simulink model "Simple_2Quad_payload_01"  (R2018b)
settings: Solver=VariableStepAuto  StartTime=0.0  StopTime=40  RelTol=1e-3
InitFcn:
  | Simple_2Quad_payload_01_const
values from neighbouring files (symbols this model uses):
  d = 1    [Simple_2Quad_payload_01_const.m]    (also in Simple_2Quad_payload_02_const.m; Simple_2Quad_payload_03_const.m; Simple_2Quad_payload_04_const.m)
  g = 9.81    [Colab_4Quad_model_01_const.m]    (also in Colab_4Quad_model_02_const.m; Simple_2Quad_payload_01_const.m; Simple_2Quad_payload_02_const.m; Simple_2Quad_payload_03_const.m)
  I = 1    [Simple_2Quad_payload_01_const.m]    (also in Simple_2Quad_payload_02_const.m; Simple_2Quad_payload_03_const.m; Simple_2Quad_payload_04_const.m)
  l2 = 1    [Simple_2Quad_payload_01_const.m]    (also in Simple_2Quad_payload_02_const.m; Simple_2Quad_payload_03_const.m)
  M = 1.0    (= 1)    [Colab_4Quad_model_01_const.m]    (also in Colab_4Quad_model_02_const.m; Simple_2Quad_payload_01_const.m; Simple_2Quad_payload_02_const.m; Simple_2Quad_payload_03_const.m)
  m1 = 1    [Simple_2Quad_payload_01_const.m]    (also in Simple_2Quad_payload_02_const.m; Simple_2Quad_payload_03_const.m)
  m2 = 1    [Simple_2Quad_payload_01_const.m]    (also in Simple_2Quad_payload_02_const.m; Simple_2Quad_payload_03_const.m)
settings Model: Creator=ali  LastModifiedBy=ali

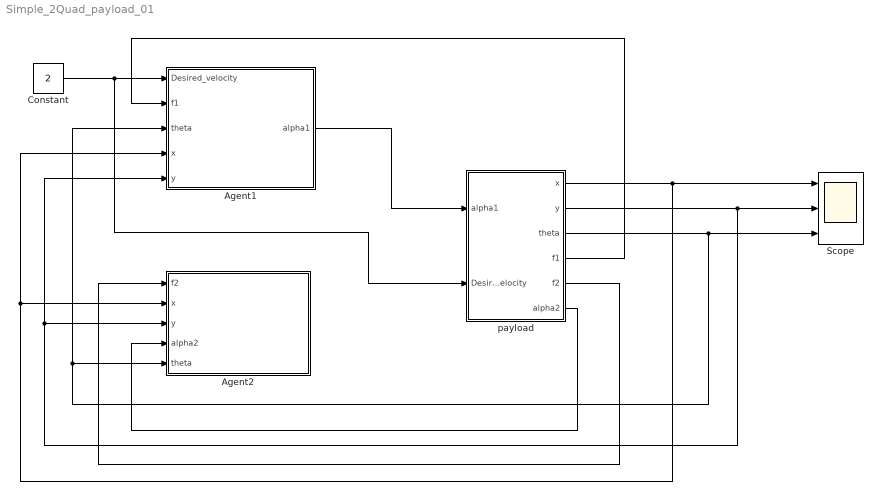
== system Simple_2Quad_payload_01 ==
  Agent1 : Subsystem
  Agent2 : Subsystem
  Constant : Constant  Value=2
  Scope : Scope  NumInputPorts=3
  payload : Subsystem
  wires:
  Constant/1 -> payload/2(Desired_velocity), Agent1/1(Desired_velocity)
  payload/3(theta) -> Scope/3, Agent2/5(theta), Agent1/3(theta)
  payload/1(x) -> Scope/1, Agent2/2(x), Agent1/4(x)
  payload/2(y) -> Scope/2, Agent2/3(y), Agent1/5(y)
  Agent1/1(alpha1) -> payload/1(alpha1)
  payload/4(f1) -> Agent1/2(f1)
  payload/5(f2) -> Agent2/1(f2)
  payload/6(alpha2) -> Agent2/4(alpha2)

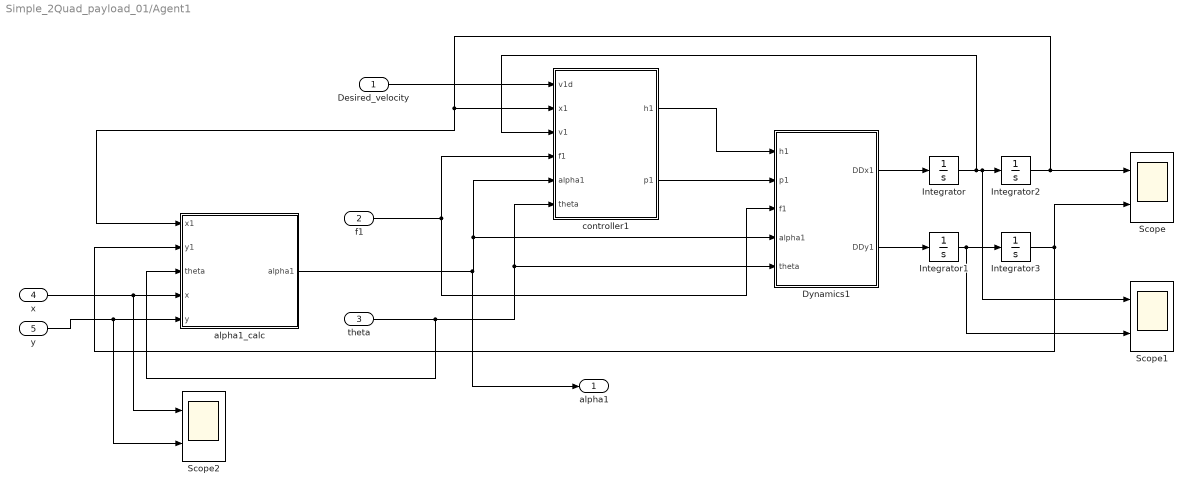
== system Simple_2Quad_payload_01/Agent1 ==
  Desired_velocity : Inport
  f1 : Inport  Port=2
  theta : Inport  Port=3
  x : Inport  Port=4
  y : Inport  Port=5
  Dynamics1 : MATLAB Function  TreatAsAtomicUnit=on
  Integrator : Integrator
  Integrator1 : Integrator
  Integrator2 : Integrator  InitialCondition=1
  Integrator3 : Integrator  InitialCondition=10
  Scope : Scope  NumInputPorts=2
  Scope1 : Scope  NumInputPorts=2
  Scope2 : Scope  NumInputPorts=2
  alpha1_calc : MATLAB Function  TreatAsAtomicUnit=on
  controller1 : Subsystem
  alpha1 : Outport
  wires:
  Dynamics1/1(DDx1) -> Integrator/1
  Dynamics1/2(DDy1) -> Integrator1/1
  Integrator/1 -> Scope1/1, Integrator2/1, controller1/3(v1)
  Integrator1/1 -> Scope1/2, Integrator3/1
  Integrator2/1 -> Scope/1, controller1/2(x1), alpha1_calc/1(x1)
  Integrator3/1 -> alpha1_calc/2(y1), Scope/2
  controller1/2(p1) -> Dynamics1/2(p1)
  controller1/1(h1) -> Dynamics1/1(h1)
  Desired_velocity/1 -> controller1/1(v1d)
  f1/1 -> controller1/4(f1), Dynamics1/3(f1)
  alpha1_calc/1(alpha1) -> alpha1/1, controller1/5(alpha1), Dynamics1/4(alpha1)
  theta/1 -> alpha1_calc/3(theta), Dynamics1/5(theta), controller1/6(theta)
  x/1 -> Scope2/1, alpha1_calc/4(x)
  y/1 -> Scope2/2, alpha1_calc/5(y)

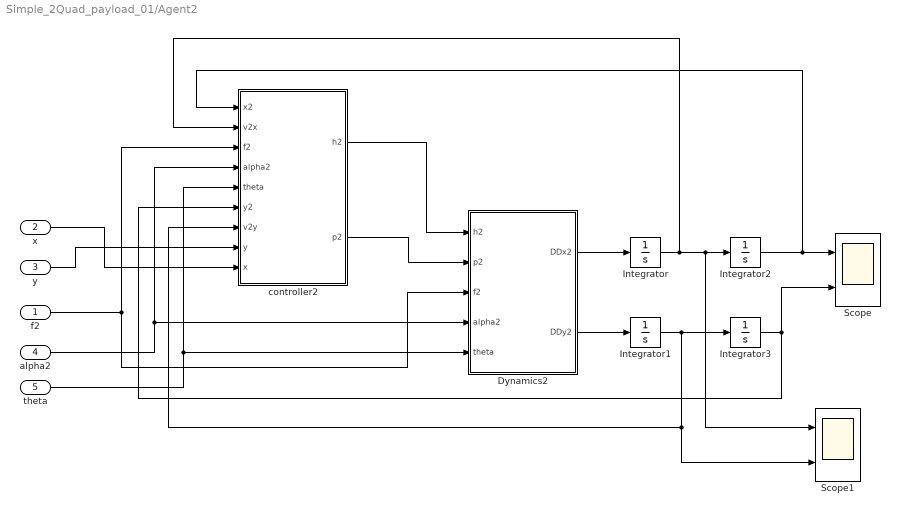
== system Simple_2Quad_payload_01/Agent2 ==
  f2 : Inport
  x : Inport  Port=2
  y : Inport  Port=3
  alpha2 : Inport  Port=4
  theta : Inport  Port=5
  Dynamics2 : MATLAB Function  TreatAsAtomicUnit=on
  Integrator : Integrator
  Integrator1 : Integrator
  Integrator2 : Integrator  InitialCondition=-1
  Integrator3 : Integrator  InitialCondition=10
  Scope : Scope  NumInputPorts=2
  Scope1 : Scope  NumInputPorts=2
  controller2 : Subsystem
  wires:
  theta/1 -> controller2/5(theta), Dynamics2/5(theta)
  alpha2/1 -> controller2/4(alpha2), Dynamics2/4(alpha2)
  f2/1 -> Dynamics2/3(f2), controller2/3(f2)
  controller2/1(h2) -> Dynamics2/1(h2)
  controller2/2(p2) -> Dynamics2/2(p2)
  Integrator3/1 -> controller2/6(y2), Scope/2
  Integrator2/1 -> controller2/1(x2), Scope/1
  Integrator1/1 -> Scope1/2, controller2/7(v2y), Integrator3/1
  Integrator/1 -> controller2/2(v2x), Scope1/1, Integrator2/1
  Dynamics2/2(DDy2) -> Integrator1/1
  Dynamics2/1(DDx2) -> Integrator/1
  y/1 -> controller2/8(y)
  x/1 -> controller2/9(x)

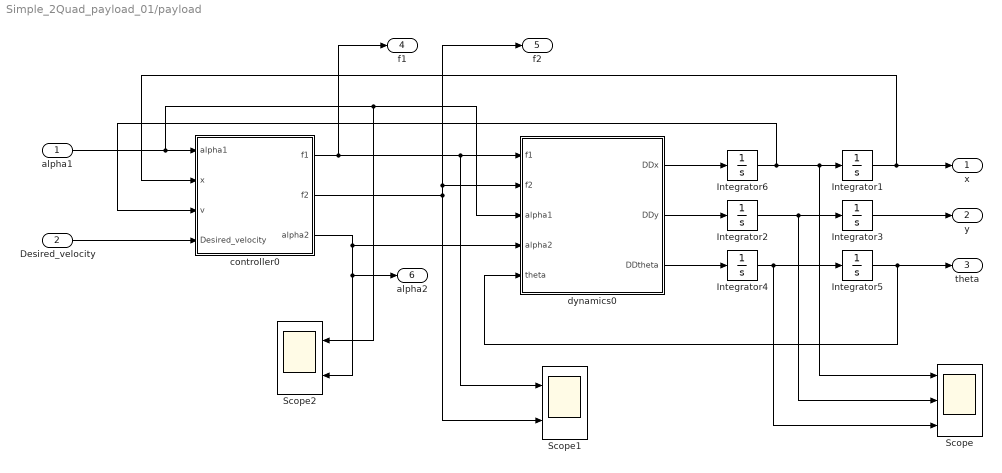
== system Simple_2Quad_payload_01/payload ==
  alpha1 : Inport
  Desired_velocity : Inport  Port=2
  Integrator{1..2,4..6} (5 alike) : Integrator
  Integrator3 : Integrator  InitialCondition=9
  Scope : Scope  NumInputPorts=3
  Scope1 : Scope  NumInputPorts=2
  Scope2 : Scope  NumInputPorts=2
  controller0 : Subsystem
  dynamics0 : MATLAB Function  TreatAsAtomicUnit=on
  x : Outport
  y : Outport  Port=2
  theta : Outport  Port=3
  f1 : Outport  Port=4
  f2 : Outport  Port=5
  alpha2 : Outport  Port=6
  wires:
  dynamics0/1(DDx) -> Integrator6/1
  dynamics0/2(DDy) -> Integrator2/1
  dynamics0/3(DDtheta) -> Integrator4/1
  Integrator4/1 -> Scope/3, Integrator5/1
  Integrator1/1 -> controller0/2(x), x/1
  Integrator3/1 -> y/1
  Integrator5/1 -> dynamics0/5(theta), theta/1
  controller0/1(f1) -> f1/1, dynamics0/1(f1), Scope1/1
  controller0/2(f2) -> f2/1, dynamics0/2(f2), Scope1/2
  controller0/3(alpha2) -> Scope2/2, alpha2/1, dynamics0/4(alpha2)
  alpha1/1 -> dynamics0/3(alpha1), Scope2/1, controller0/1(alpha1)
  Desired_velocity/1 -> controller0/4(Desired_velocity)
  Integrator2/1 -> Scope/2, Integrator3/1
  Integrator6/1 -> controller0/3(v), Scope/1, Integrator1/1

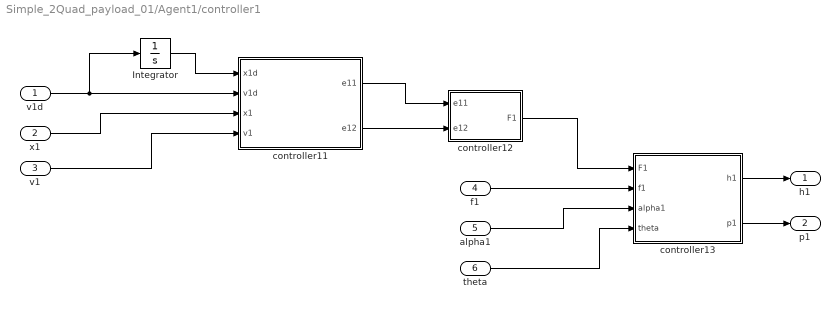
== system Simple_2Quad_payload_01/Agent1/controller1 ==
  v1d : Inport
  x1 : Inport  Port=2
  v1 : Inport  Port=3
  f1 : Inport  Port=4
  alpha1 : Inport  Port=5
  theta : Inport  Port=6
  Integrator : Integrator
  controller11 : MATLAB Function  TreatAsAtomicUnit=on
  controller12 : MATLAB Function  TreatAsAtomicUnit=on
  controller13 : MATLAB Function  TreatAsAtomicUnit=on
  h1 : Outport
  p1 : Outport  Port=2
  wires:
  controller11/1(e11) -> controller12/1(e11)
  controller11/2(e12) -> controller12/2(e12)
  controller12/1(F1) -> controller13/1(F1)
  controller13/1(h1) -> h1/1
  controller13/2(p1) -> p1/1
  v1d/1 -> Integrator/1, controller11/2(v1d)
  Integrator/1 -> controller11/1(x1d)
  x1/1 -> controller11/3(x1)
  v1/1 -> controller11/4(v1)
  f1/1 -> controller13/2(f1)
  alpha1/1 -> controller13/3(alpha1)
  theta/1 -> controller13/4(theta)

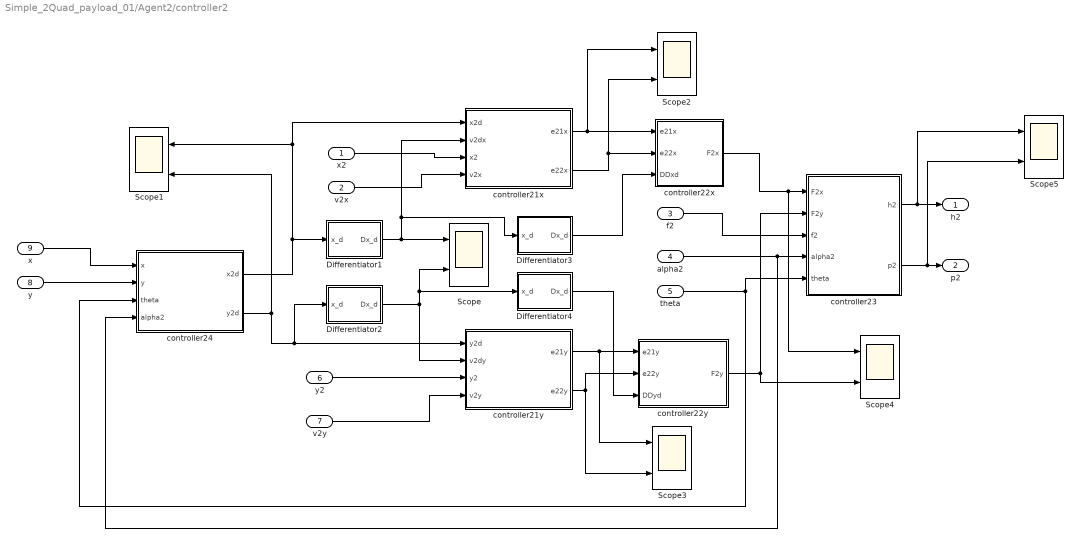
== system Simple_2Quad_payload_01/Agent2/controller2 ==
  x2 : Inport
  v2x : Inport  Port=2
  f2 : Inport  Port=3
  alpha2 : Inport  Port=4
  theta : Inport  Port=5
  y2 : Inport  Port=6
  v2y : Inport  Port=7
  y : Inport  Port=8
  x : Inport  Port=9
  Differentiator1 : Subsystem
  Differentiator2 : Subsystem
  Differentiator3 : Subsystem
  Differentiator4 : Subsystem
  Scope{,1..5} (6 alike) : Scope  NumInputPorts=2
  controller21x : MATLAB Function  TreatAsAtomicUnit=on
  controller21y : MATLAB Function  TreatAsAtomicUnit=on
  controller22x : MATLAB Function  TreatAsAtomicUnit=on
  controller22y : MATLAB Function  TreatAsAtomicUnit=on
  controller23 : MATLAB Function  TreatAsAtomicUnit=on
  controller24 : MATLAB Function  TreatAsAtomicUnit=on
  h2 : Outport
  p2 : Outport  Port=2
  wires:
  theta/1 -> controller24/3(theta), controller23/5(theta)
  alpha2/1 -> controller24/4(alpha2), controller23/4(alpha2)
  f2/1 -> controller23/3(f2)
  v2x/1 -> controller21x/4(v2x)
  x2/1 -> controller21x/3(x2)
  controller23/2(p2) -> Scope5/2, p2/1
  controller22x/1(F2x) -> Scope4/1, controller23/1(F2x)
  controller21x/1(e21x) -> Scope2/1, controller22x/1(e21x)
  controller21y/1(e21y) -> controller22y/1(e21y), Scope3/1
  controller22y/1(F2y) -> Scope4/2, controller23/2(F2y)
  y2/1 -> controller21y/3(y2)
  v2y/1 -> controller21y/4(v2y)
  controller24/1(x2d) -> Differentiator1/1(x_d), Scope1/1, controller21x/1(x2d)
  controller24/2(y2d) -> Differentiator2/1(x_d), controller21y/1(y2d), Scope1/2
  y/1 -> controller24/2(y)
  x/1 -> controller24/1(x)
  Differentiator1/1(Dx_d) -> Scope/1, Differentiator3/1(x_d), controller21x/2(v2dx)
  Differentiator2/1(Dx_d) -> Differentiator4/1(x_d), Scope/2, controller21y/2(v2dy)
  controller21x/2(e22x) -> Scope2/2, controller22x/2(e22x)
  controller21y/2(e22y) -> Scope3/2, controller22y/2(e22y)
  controller23/1(h2) -> Scope5/1, h2/1
  Differentiator3/1(Dx_d) -> controller22x/3(DDxd)
  Differentiator4/1(Dx_d) -> controller22y/3(DDyd)

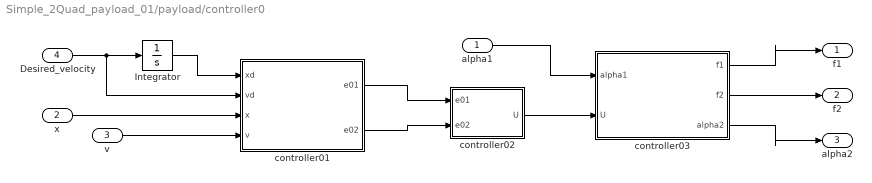
== system Simple_2Quad_payload_01/payload/controller0 ==
  alpha1 : Inport
  x : Inport  Port=2
  v : Inport  Port=3
  Desired_velocity : Inport  Port=4
  Integrator : Integrator
  controller01 : MATLAB Function  TreatAsAtomicUnit=on
  controller02 : MATLAB Function  TreatAsAtomicUnit=on
  controller03 : MATLAB Function  TreatAsAtomicUnit=on
  f1 : Outport
  f2 : Outport  Port=2
  alpha2 : Outport  Port=3
  wires:
  controller03/2(f2) -> f2/1
  controller03/1(f1) -> f1/1
  controller03/3(alpha2) -> alpha2/1
  alpha1/1 -> controller03/1(alpha1)
  x/1 -> controller01/3(x)
  controller01/2(e02) -> controller02/2(e02)
  controller01/1(e01) -> controller02/1(e01)
  v/1 -> controller01/4(v)
  Integrator/1 -> controller01/1(xd)
  Desired_velocity/1 -> controller01/2(vd), Integrator/1
  controller02/1(U) -> controller03/2(U)

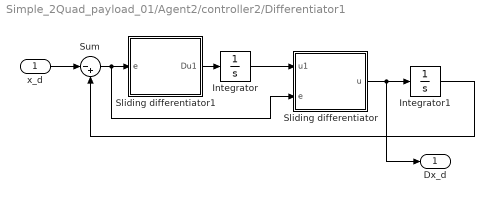
== system Simple_2Quad_payload_01/Agent2/controller2/Differentiator1 ==
  x_d : Inport
  Integrator : Integrator  InitialCondition=1
  Integrator1 : Integrator  InitialCondition=1
  Sliding differentiator : MATLAB Function  TreatAsAtomicUnit=on
  Sliding differentiator1 : MATLAB Function  TreatAsAtomicUnit=on
  Sum : Sum  Inputs=|-+
  Dx_d : Outport
  wires:
  Sliding differentiator/1(u) -> Integrator1/1, Dx_d/1
  Sliding differentiator1/1(Du1) -> Integrator/1
  Integrator/1 -> Sliding differentiator/1(u1)
  x_d/1 -> Sum/1
  Sum/1 -> Sliding differentiator/2(e), Sliding differentiator1/1(e)
  Integrator1/1 -> Sum/2

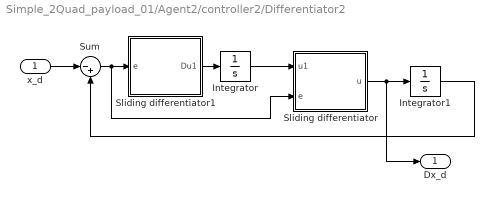
== system Simple_2Quad_payload_01/Agent2/controller2/Differentiator2 ==
  x_d : Inport
  Integrator : Integrator  InitialCondition=1
  Integrator1 : Integrator  InitialCondition=1
  Sliding differentiator : MATLAB Function  TreatAsAtomicUnit=on
  Sliding differentiator1 : MATLAB Function  TreatAsAtomicUnit=on
  Sum : Sum  Inputs=|-+
  Dx_d : Outport
  wires:
  Integrator1/1 -> Sum/2
  Sum/1 -> Sliding differentiator1/1(e), Sliding differentiator/2(e)
  x_d/1 -> Sum/1
  Integrator/1 -> Sliding differentiator/1(u1)
  Sliding differentiator1/1(Du1) -> Integrator/1
  Sliding differentiator/1(u) -> Dx_d/1, Integrator1/1

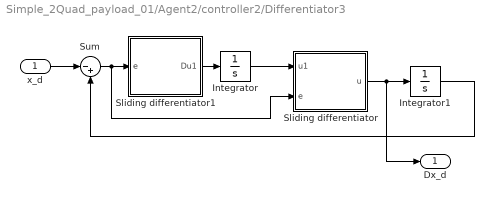
== system Simple_2Quad_payload_01/Agent2/controller2/Differentiator3 ==
  x_d : Inport
  Integrator : Integrator  InitialCondition=1
  Integrator1 : Integrator  InitialCondition=1
  Sliding differentiator : MATLAB Function  TreatAsAtomicUnit=on
  Sliding differentiator1 : MATLAB Function  TreatAsAtomicUnit=on
  Sum : Sum  Inputs=|-+
  Dx_d : Outport
  wires:
  Integrator1/1 -> Sum/2
  Sum/1 -> Sliding differentiator1/1(e), Sliding differentiator/2(e)
  x_d/1 -> Sum/1
  Integrator/1 -> Sliding differentiator/1(u1)
  Sliding differentiator1/1(Du1) -> Integrator/1
  Sliding differentiator/1(u) -> Dx_d/1, Integrator1/1

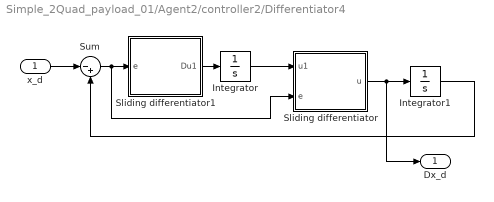
== system Simple_2Quad_payload_01/Agent2/controller2/Differentiator4 ==
  x_d : Inport
  Integrator : Integrator  InitialCondition=1
  Integrator1 : Integrator  InitialCondition=1
  Sliding differentiator : MATLAB Function  TreatAsAtomicUnit=on
  Sliding differentiator1 : MATLAB Function  TreatAsAtomicUnit=on
  Sum : Sum  Inputs=|-+
  Dx_d : Outport
  wires:
  Sliding differentiator/1(u) -> Integrator1/1, Dx_d/1
  Sliding differentiator1/1(Du1) -> Integrator/1
  Integrator/1 -> Sliding differentiator/1(u1)
  x_d/1 -> Sum/1
  Sum/1 -> Sliding differentiator/2(e), Sliding differentiator1/1(e)
  Integrator1/1 -> Sum/2

== matlab function Simple_2Quad_payload_01/Agent1/controller1/controller12 ==
  data: e11 input; F1 output; e12 input
function F1 = fcn(e11,e12)

k11 = 1;
k12 = 1;

F1 = k12*e12 - (k11^2)*e11;

end

== matlab function Simple_2Quad_payload_01/Agent1/Dynamics1 ==
  data: h1 input; DDx1 output; p1 input; f1 input; alpha1 input; theta input; DDy1 output; g parameter; m1 parameter
function [DDx1,DDy1] = fcn(h1,p1,f1,alpha1,theta,g, m1)

DDx1 = (1/m1) * (h1 - f1*cos(alpha1+theta));
DDy1 = (1/m1) * (p1 - m1*g - f1*sin(alpha1+theta));

end

== matlab function Simple_2Quad_payload_01/Agent1/controller1/controller11 ==
  data: x1d input; e11 output; v1d input; x1 input; v1 input; e12 output
function [e11,e12] = fcn(x1d,v1d,x1,v1)

k11 = 1;

e11 = x1d - x1;
u1 = v1d + k11*e11;
e12 = u1 - v1;

end

== matlab function Simple_2Quad_payload_01/Agent1/controller1/controller13 ==
  data: F1 input; h1 output; f1 input; alpha1 input; theta input; p1 output; m1 parameter; g parameter
function [h1,p1] = fcn(F1,f1,alpha1,theta,m1, g)

h1 = F1 + f1*cos(alpha1+theta);
p1 = m1*g + f1*sin(alpha1+theta);

end

== matlab function Simple_2Quad_payload_01/Agent2/Dynamics2 ==
  data: h2 input; DDx2 output; p2 input; f2 input; alpha2 input; theta input; DDy2 output; g parameter; m2 parameter
function [DDx2,DDy2] = fcn(h2,p2,f2,alpha2,theta,g, m2)

DDx2 = (1/m2) * (h2 - f2*cos(alpha2+theta));
DDy2 = (1/m2) * (p2 - m2*g - f2*sin(alpha2+theta));

end

== matlab function Simple_2Quad_payload_01/Agent2/controller2/controller22x ==
  data: e21x input; F2x output; e22x input; DDxd input
function F2x = fcn(e21x,e22x,DDxd)

k21x = 1;
k22x = 10;

F2x = DDxd + k21x*e21x + k22x*e22x;

end

== matlab function Simple_2Quad_payload_01/Agent2/controller2/controller21x ==
  data: x2d input; e21x output; v2dx input; x2 input; v2x input; e22x output
function [e21x,e22x] = fcn(x2d,v2dx,x2,v2x)

k21x = 1;

e21x = x2d - x2;
u2x = v2dx + k21x*e21x;
e22x = u2x - v2x;

end

== matlab function Simple_2Quad_payload_01/Agent2/controller2/controller23 ==
  data: F2x input; F2y input; h2 output; f2 input; alpha2 input; theta input; p2 output; m2 parameter; g parameter
function [h2,p2] = fcn(F2x,F2y,f2,alpha2,theta,m2, g)

h2 = F2x + f2*cos(alpha2+theta);
p2 = F2y + m2*g + f2*sin(alpha2+theta);

end

== matlab function Simple_2Quad_payload_01/payload/dynamics0 ==
  data: f1 input; DDx output; f2 input; alpha1 input; alpha2 input; theta input; DDy output; DDtheta output; M parameter; g parameter; d parameter; I parameter
function [DDx,DDy,DDtheta] = fcn(f1,f2,alpha1,alpha2,theta,M, g, d, I)

DDx = (1/M) * ( f1*cos(alpha1+theta) + f2*cos(alpha2+theta) );
DDy = (1/M) * ( f1*sin(alpha1+theta) + f2*sin(alpha2+theta) - M*g );
DDtheta = (d/I) * ( f1*sin(alpha1) - f2*sin(alpha2) );

end

== matlab function Simple_2Quad_payload_01/payload/controller0/controller03 ==
  data: alpha1 input; f1 output; U input; f2 output; alpha2 output; M parameter; g parameter
function [f1,f2,alpha2] = fcn(alpha1,U,M, g)

f1 = M*g/2/sin(alpha1);
alpha2 = abs( atan( (M*g/2) / (U - f1*cos(alpha1)) ) );
f2 = M*g/2/sin(alpha2);

end

== matlab function Simple_2Quad_payload_01/Agent1/alpha1_calc ==
  data: x1 input; alpha1 output; y1 input; theta input; d parameter; x input; y input
function alpha1 = fcn(x1,y1,theta,d, x, y)

alpha1 = abs( atan( (y1 - y - d*sin(theta)) / (x1 - x - d*cos(theta)) ) );

end

== matlab function Simple_2Quad_payload_01/Agent2/controller2/controller21y ==
  data: y2d input; e21y output; v2dy input; y2 input; v2y input; e22y output
function [e21y,e22y] = fcn(y2d,v2dy,y2,v2y)

k21y = 1;

e21y = y2d - y2;
u2y = v2dy + k21y*e21y;
e22y = u2y - v2y;

end

== matlab function Simple_2Quad_payload_01/Agent2/controller2/controller22y ==
  data: e21y input; F2y output; e22y input; DDyd input
function F2y = fcn(e21y,e22y,DDyd)

k21y = 1;
k22y = 10;

F2y = DDyd + k21y*e21y + k22y*e22y;

end

== matlab function Simple_2Quad_payload_01/Agent2/controller2/controller24 ==
  data: x input; x2d output; y input; theta input; y2d output; alpha2 input; d parameter; l2 parameter
function [x2d,y2d] = fcn(x,y,theta,alpha2, d, l2)

x2d = x - d*cos(theta) + l2*cos(alpha2+theta);
y2d = y - d*sin(theta) + l2*sin(alpha2+theta);

end

== matlab function Simple_2Quad_payload_01/payload/controller0/controller01 ==
  data: xd input; e01 output; vd input; x input; v input; e02 output
function [e01,e02] = fcn(xd,vd,x,v)

k01 = 1;

e01 = xd - x;
u0 = vd + k01*e01;
e02 = u0 - v;

end

== matlab function Simple_2Quad_payload_01/payload/controller0/controller02 ==
  data: e01 input; U output; e02 input
function U = fcn(e01,e02)

k01 = 1;
k02 = 1;

U = k02*e02 - (k01^2)*e01;

end

== matlab function Simple_2Quad_payload_01/Agent2/controller2/Differentiator1/Sliding differentiator ==
  data: u output; u1 input; e input
function u = fcn(u1,e)

b=1;

ABS = abs(e);
SGN = e ./ (ABS + 0.01);
u = u1 - b*((ABS.^0.5).*SGN); 

end

== matlab function Simple_2Quad_payload_01/Agent2/controller2/Differentiator1/Sliding differentiator1 ==
  data: Du1 output; e input
function Du1 = fcn(e)

a=1;

ABS = abs(e);
SGN = e ./ (ABS + 0.01);
Du1 = - a*SGN;

end

== matlab function Simple_2Quad_payload_01/Agent2/controller2/Differentiator2/Sliding differentiator ==
  data: u output; u1 input; e input
function u = fcn(u1,e)

b=1;

ABS = abs(e);
SGN = e ./ (ABS + 0.01);
u = u1 - b*((ABS.^0.5).*SGN); 

end

== matlab function Simple_2Quad_payload_01/Agent2/controller2/Differentiator2/Sliding differentiator1 ==
  data: Du1 output; e input
function Du1 = fcn(e)

a=1;

ABS = abs(e);
SGN = e ./ (ABS + 0.01);
Du1 = - a*SGN;

end

== matlab function Simple_2Quad_payload_01/Agent2/controller2/Differentiator3/Sliding differentiator ==
  data: u output; u1 input; e input
function u = fcn(u1,e)

b=1;

ABS = abs(e);
SGN = e ./ (ABS + 0.01);
u = u1 - b*((ABS.^0.5).*SGN); 

end

== matlab function Simple_2Quad_payload_01/Agent2/controller2/Differentiator3/Sliding differentiator1 ==
  data: Du1 output; e input
function Du1 = fcn(e)

a=1;

ABS = abs(e);
SGN = e ./ (ABS + 0.01);
Du1 = - a*SGN;

end

== matlab function Simple_2Quad_payload_01/Agent2/controller2/Differentiator4/Sliding differentiator ==
  data: u output; u1 input; e input
function u = fcn(u1,e)

b=1;

ABS = abs(e);
SGN = e ./ (ABS + 0.01);
u = u1 - b*((ABS.^0.5).*SGN); 

end

== matlab function Simple_2Quad_payload_01/Agent2/controller2/Differentiator4/Sliding differentiator1 ==
  data: Du1 output; e input
function Du1 = fcn(e)

a=1;

ABS = abs(e);
SGN = e ./ (ABS + 0.01);
Du1 = - a*SGN;

end
